simulink model "cv5model"  (R2022b)
settings: Solver=ode45  StartTime=0.0  StopTime=1  MaxStep=.001  RelTol=1e-3  AbsTol=1e-3  EnableMultiTasking=on
values from neighbouring files (symbols this model uses):
  cpr = 4186    [cv5par.m]
  l12r = 1.02e6    (= 1020000)    [cv5par.m]
  S1ir = S1r/nr    (= 0.377)    [cv5par.m]
  Ti1r = 90    [cv5par.m]
  Ti2r = 20    [cv5par.m]
settings Model: Creator=EM  LastModifiedBy=EM
settings DataIOCC: SaveFormat=Array  SignalLoggingSaveFormat=ModelDataLogs  SaveOutput=off  ReturnWorkspaceOutputs=off  TimeSaveName=t
settings OptimizationCC: BlockReduction=off  BooleanDataType=off  InitFltsAndDblsToZero=on
settings DebuggingCC: SaveWithParameterizedLinksMsg=none  UnderspecifiedInitializationDetection=Classic  MergeDetectMultiDrivingBlocksExec=none  SignalResolutionControl=TryResolveAllWithWarning  MultiTaskCondExecSysMsg=none  UnconnectedInputMsg=warning  UnconnectedOutputMsg=warning  UnconnectedLineMsg=warning
settings HardwareCC: ProdBitPerPointer=32  ProdBitPerSizeT=32  ProdBitPerPtrDiffT=32  ProdLargestAtomicFloat=None  ProdIntDivRoundTo=Undefined  ProdEndianess=Unspecified  ProdWordSize=32  ProdHWDeviceType=32-bit Generic  TargetUnknown=on
settings ModelReferenceCC: PropagateSignalLabelsOutOfModel=off
settings GRTTargetCC: TargetFcnLib=ansi_tfl_tmw.mat  TargetLangStandard=C89/C90 (ANSI)  CombineOutputUpdateFcns=off  GRTInterface=on
settings ConfigComp: CovMetricSettings=dw  CovSaveCumulativeToWorkspaceVar=on  CovSaveSingleToWorkspaceVar=on

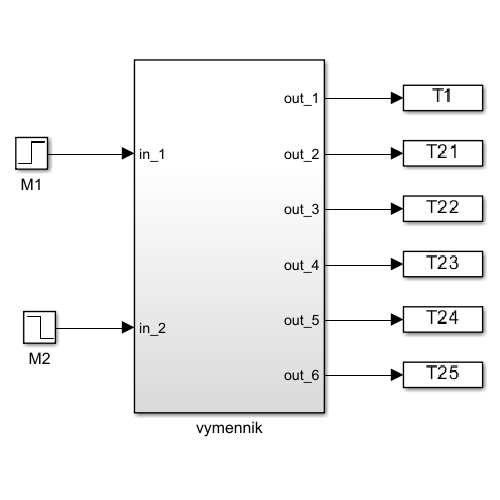
[thumbnail: Simulink's stored preview of the top-level diagram]
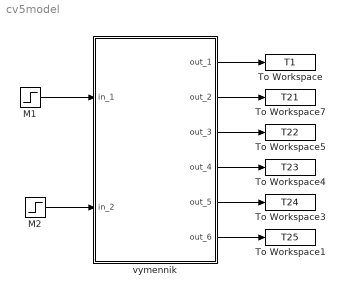
== system cv5model ==
  M1 : Step  Time=0.5  Before=500  After=500  SampleTime=0
  M2 : Step  Time=0.5  Before=500  After=250  SampleTime=0
  To Workspace : ToWorkspace  VariableName=T1
      settings: MaxDataPoints=20000
  To Workspace1 : ToWorkspace  VariableName=T25
      settings: MaxDataPoints=20000
  To Workspace3 : ToWorkspace  VariableName=T24
      settings: MaxDataPoints=20000
  To Workspace4 : ToWorkspace  VariableName=T23
      settings: MaxDataPoints=20000
  To Workspace5 : ToWorkspace  VariableName=T22
      settings: MaxDataPoints=20000
  To Workspace7 : ToWorkspace  VariableName=T21
      settings: MaxDataPoints=20000
  vymennik : Subsystem
  wires:
  M2/1 -> vymennik/2(in_2)
  M1/1 -> vymennik/1(in_1)
  vymennik/1(out_1) -> To Workspace/1
  vymennik/2(out_2) -> To Workspace7/1
  vymennik/3(out_3) -> To Workspace5/1
  vymennik/4(out_4) -> To Workspace4/1
  vymennik/5(out_5) -> To Workspace3/1
  vymennik/6(out_6) -> To Workspace1/1

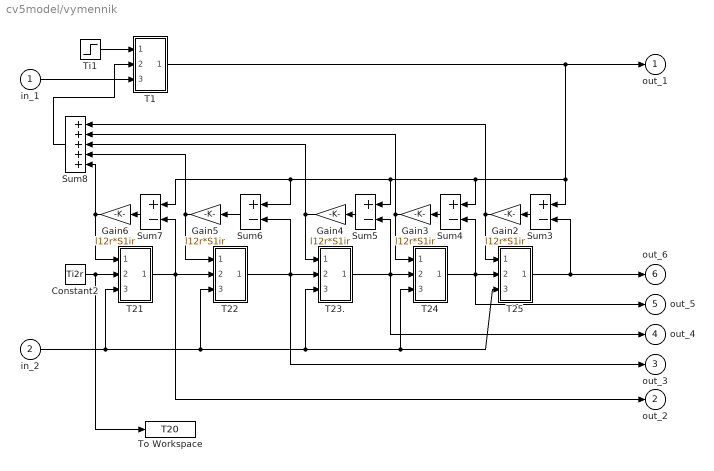
== system cv5model/vymennik ==
  in_1 : Inport
  in_2 : Inport  Port=2
  Constant2 : Constant  Value=Ti2r
  Gain{2..6} (5 alike) : Gain  Gain=l12r*S1ir  SaturateOnIntegerOverflow=on  OutDataTypeStr=Inherit: Same as input  ParamDataTypeStr=Inherit: Same as input
  Sum{3..7} (5 alike) : Sum  Inputs=+-  InputSameDT=on  SaturateOnIntegerOverflow=on  OutDataTypeStr=Inherit: Same as first input
  Sum8 : Sum  Inputs=+++++  InputSameDT=on  SaturateOnIntegerOverflow=on  OutDataTypeStr=Inherit: Same as first input
  T1 : Subsystem
  T21 : Subsystem
  T22 : Subsystem
  T23. : Subsystem
  T24 : Subsystem
  T25 : Subsystem
  Ti1 : Step  Time=0  After=Ti1r  SampleTime=0
  To Workspace : ToWorkspace  VariableName=T20
      settings: MaxDataPoints=20000
  out_1 : Outport
  out_2 : Outport  Port=2
  out_3 : Outport  Port=3
  out_4 : Outport  Port=4
  out_5 : Outport  Port=5
  out_6 : Outport  Port=6
  wires:
  T25/1(out_1) -> out_6/1, Sum3/2
  Sum8/1 -> T1/2(in_2)
  Gain6/1 -> Sum8/5, T21/1(in_1)
  T1/1(out_1) -> out_1/1, Sum3/1, Sum4/1, Sum5/1, Sum6/1, Sum7/1
  Gain5/1 -> Sum8/4, T22/1(in_1)
  Gain4/1 -> Sum8/3, T23./1(in_1)
  Gain3/1 -> Sum8/2, T24/1(in_1)
  Sum7/1 -> Gain6/1
  Sum6/1 -> Gain5/1
  Sum5/1 -> Gain4/1
  Sum4/1 -> Gain3/1
  Gain2/1 -> Sum8/1, T25/1(in_1)
  Constant2/1 -> T21/2(in_2), To Workspace/1
  in_2/1 -> T21/3(in_3), T23./3(in_3), T24/3(in_3), T25/3(in_3), T22/3(in_3)
  Sum3/1 -> Gain2/1
  Ti1/1 -> T1/1(in_1)
  in_1/1 -> T1/3(in_3)
  T21/1(out_1) -> out_2/1, T22/2(in_2), Sum7/2
  T22/1(out_1) -> out_3/1, T23./2(in_2), Sum6/2
  T23./1(out_1) -> out_4/1, T24/2(in_2), Sum5/2
  T24/1(out_1) -> out_5/1, T25/2(in_2), Sum4/2

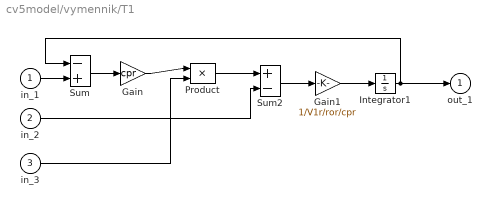
== system cv5model/vymennik/T1 ==
  in_1 : Inport
  in_2 : Inport  Port=2
  in_3 : Inport  Port=3
  Gain : Gain  Gain=cpr  SaturateOnIntegerOverflow=on  OutDataTypeStr=Inherit: Same as input  ParamDataTypeStr=Inherit: Same as input
  Gain1 : Gain  Gain=1/V1r/ror/cpr  SaturateOnIntegerOverflow=on  OutDataTypeStr=Inherit: Same as input  ParamDataTypeStr=Inherit: Same as input
  Integrator1 : Integrator  InitialCondition=20
  Product : Product  InputSameDT=on  RndMeth=Zero  SaturateOnIntegerOverflow=on  OutDataTypeStr=Inherit: Same as first input
  Sum : Sum  Inputs=-+  InputSameDT=on  SaturateOnIntegerOverflow=on  OutDataTypeStr=Inherit: Same as first input
  Sum2 : Sum  Inputs=+-  InputSameDT=on  SaturateOnIntegerOverflow=on  OutDataTypeStr=Inherit: Same as first input
  out_1 : Outport
  wires:
  Gain1/1 -> Integrator1/1
  Sum2/1 -> Gain1/1
  Sum/1 -> Gain/1
  in_1/1 -> Sum/2
  Integrator1/1 -> Sum/1, out_1/1
  in_2/1 -> Sum2/2
  Product/1 -> Sum2/1
  Gain/1 -> Product/1
  in_3/1 -> Product/2

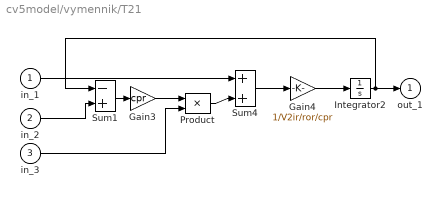
== system cv5model/vymennik/T21 ==
  in_1 : Inport
  in_2 : Inport  Port=2
  in_3 : Inport  Port=3
  Gain3 : Gain  Gain=cpr  SaturateOnIntegerOverflow=on  OutDataTypeStr=Inherit: Same as input  ParamDataTypeStr=Inherit: Same as input
  Gain4 : Gain  Gain=1/V2ir/ror/cpr  SaturateOnIntegerOverflow=on  OutDataTypeStr=Inherit: Same as input  ParamDataTypeStr=Inherit: Same as input
  Integrator2 : Integrator  InitialCondition=20
  Product : Product  InputSameDT=on  RndMeth=Zero  SaturateOnIntegerOverflow=on  OutDataTypeStr=Inherit: Same as first input
  Sum1 : Sum  Inputs=-+  InputSameDT=on  SaturateOnIntegerOverflow=on  OutDataTypeStr=Inherit: Same as first input
  Sum4 : Sum  InputSameDT=on  SaturateOnIntegerOverflow=on  OutDataTypeStr=Inherit: Same as first input
  out_1 : Outport
  wires:
  Product/1 -> Sum4/2
  Gain3/1 -> Product/1
  Gain4/1 -> Integrator2/1
  Sum4/1 -> Gain4/1
  Sum1/1 -> Gain3/1
  in_1/1 -> Sum4/1
  Integrator2/1 -> Sum1/1, out_1/1
  in_2/1 -> Sum1/2
  in_3/1 -> Product/2

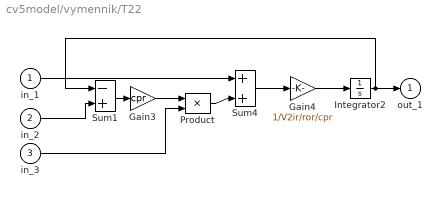
== system cv5model/vymennik/T22 ==
  in_1 : Inport
  in_2 : Inport  Port=2
  in_3 : Inport  Port=3
  Gain3 : Gain  Gain=cpr  SaturateOnIntegerOverflow=on  OutDataTypeStr=Inherit: Same as input  ParamDataTypeStr=Inherit: Same as input
  Gain4 : Gain  Gain=1/V2ir/ror/cpr  SaturateOnIntegerOverflow=on  OutDataTypeStr=Inherit: Same as input  ParamDataTypeStr=Inherit: Same as input
  Integrator2 : Integrator  InitialCondition=20
  Product : Product  InputSameDT=on  RndMeth=Zero  SaturateOnIntegerOverflow=on  OutDataTypeStr=Inherit: Same as first input
  Sum1 : Sum  Inputs=-+  InputSameDT=on  SaturateOnIntegerOverflow=on  OutDataTypeStr=Inherit: Same as first input
  Sum4 : Sum  InputSameDT=on  SaturateOnIntegerOverflow=on  OutDataTypeStr=Inherit: Same as first input
  out_1 : Outport
  wires:
  in_3/1 -> Product/2
  in_2/1 -> Sum1/2
  in_1/1 -> Sum4/1
  Sum1/1 -> Gain3/1
  Sum4/1 -> Gain4/1
  Gain4/1 -> Integrator2/1
  Integrator2/1 -> out_1/1, Sum1/1
  Gain3/1 -> Product/1
  Product/1 -> Sum4/2

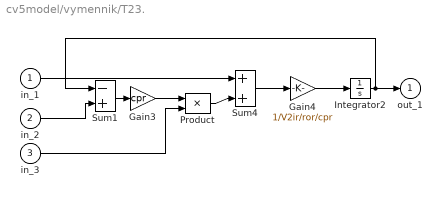
== system cv5model/vymennik/T23. ==
  in_1 : Inport
  in_2 : Inport  Port=2
  in_3 : Inport  Port=3
  Gain3 : Gain  Gain=cpr  SaturateOnIntegerOverflow=on  OutDataTypeStr=Inherit: Same as input  ParamDataTypeStr=Inherit: Same as input
  Gain4 : Gain  Gain=1/V2ir/ror/cpr  SaturateOnIntegerOverflow=on  OutDataTypeStr=Inherit: Same as input  ParamDataTypeStr=Inherit: Same as input
  Integrator2 : Integrator  InitialCondition=20
  Product : Product  InputSameDT=on  RndMeth=Zero  SaturateOnIntegerOverflow=on  OutDataTypeStr=Inherit: Same as first input
  Sum1 : Sum  Inputs=-+  InputSameDT=on  SaturateOnIntegerOverflow=on  OutDataTypeStr=Inherit: Same as first input
  Sum4 : Sum  InputSameDT=on  SaturateOnIntegerOverflow=on  OutDataTypeStr=Inherit: Same as first input
  out_1 : Outport
  wires:
  Product/1 -> Sum4/2
  Gain3/1 -> Product/1
  Gain4/1 -> Integrator2/1
  Sum4/1 -> Gain4/1
  Sum1/1 -> Gain3/1
  in_1/1 -> Sum4/1
  Integrator2/1 -> Sum1/1, out_1/1
  in_2/1 -> Sum1/2
  in_3/1 -> Product/2

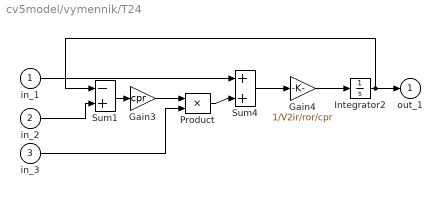
== system cv5model/vymennik/T24 ==
  in_1 : Inport
  in_2 : Inport  Port=2
  in_3 : Inport  Port=3
  Gain3 : Gain  Gain=cpr  SaturateOnIntegerOverflow=on  OutDataTypeStr=Inherit: Same as input  ParamDataTypeStr=Inherit: Same as input
  Gain4 : Gain  Gain=1/V2ir/ror/cpr  SaturateOnIntegerOverflow=on  OutDataTypeStr=Inherit: Same as input  ParamDataTypeStr=Inherit: Same as input
  Integrator2 : Integrator  InitialCondition=20
  Product : Product  InputSameDT=on  RndMeth=Zero  SaturateOnIntegerOverflow=on  OutDataTypeStr=Inherit: Same as first input
  Sum1 : Sum  Inputs=-+  InputSameDT=on  SaturateOnIntegerOverflow=on  OutDataTypeStr=Inherit: Same as first input
  Sum4 : Sum  InputSameDT=on  SaturateOnIntegerOverflow=on  OutDataTypeStr=Inherit: Same as first input
  out_1 : Outport
  wires:
  in_3/1 -> Product/2
  in_2/1 -> Sum1/2
  in_1/1 -> Sum4/1
  Sum1/1 -> Gain3/1
  Sum4/1 -> Gain4/1
  Gain4/1 -> Integrator2/1
  Integrator2/1 -> out_1/1, Sum1/1
  Gain3/1 -> Product/1
  Product/1 -> Sum4/2

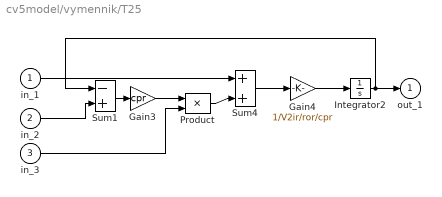
== system cv5model/vymennik/T25 ==
  in_1 : Inport
  in_2 : Inport  Port=2
  in_3 : Inport  Port=3
  Gain3 : Gain  Gain=cpr  SaturateOnIntegerOverflow=on  OutDataTypeStr=Inherit: Same as input  ParamDataTypeStr=Inherit: Same as input
  Gain4 : Gain  Gain=1/V2ir/ror/cpr  SaturateOnIntegerOverflow=on  OutDataTypeStr=Inherit: Same as input  ParamDataTypeStr=Inherit: Same as input
  Integrator2 : Integrator  InitialCondition=20
  Product : Product  InputSameDT=on  RndMeth=Zero  SaturateOnIntegerOverflow=on  OutDataTypeStr=Inherit: Same as first input
  Sum1 : Sum  Inputs=-+  InputSameDT=on  SaturateOnIntegerOverflow=on  OutDataTypeStr=Inherit: Same as first input
  Sum4 : Sum  InputSameDT=on  SaturateOnIntegerOverflow=on  OutDataTypeStr=Inherit: Same as first input
  out_1 : Outport
  wires:
  Product/1 -> Sum4/2
  Gain3/1 -> Product/1
  Gain4/1 -> Integrator2/1
  Sum4/1 -> Gain4/1
  Sum1/1 -> Gain3/1
  in_1/1 -> Sum4/1
  Integrator2/1 -> Sum1/1, out_1/1
  in_2/1 -> Sum1/2
  in_3/1 -> Product/2
